simulink model "ASV1_P_RobotMobile1D"  (R2023b)
settings: Solver=VariableStepAuto  StartTime=0.0  StopTime=30  RelTol=1e-3
libraries: simulink x1
settings Model: Creator=LENOVO  LastModifiedBy=LENOVO

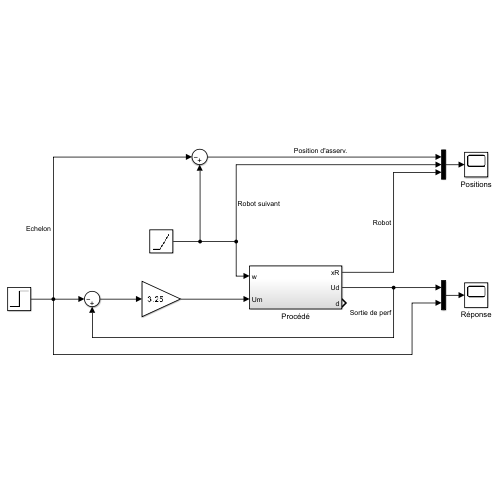
[thumbnail: Simulink's stored preview of the top-level diagram]
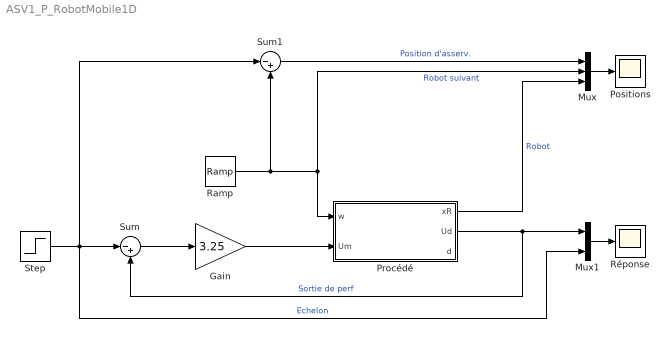
== system ASV1_P_RobotMobile1D ==
  Gain : Gain  Gain=3.25
  Mux : Mux  Inputs=3
  Mux1 : Mux  Inputs=2
  Positions : Scope
  Procédé : Subsystem
  Ramp : simulink/Sources/Ramp  slope=0.5  start=10  InitialOutput=0
  Réponse : Scope
  Step : Step  Time=0  After=0.25  SampleTime=0
  Sum : Sum  Inputs=|-+
  Sum1 : Sum  Inputs=|-+
  wires:
  Step/1 -> Mux1/2, Sum1/1, Sum/1  "Echelon"
  Sum/1 -> Gain/1
  Ramp/1 -> Mux/2, Procédé/1(w), Sum1/2  "Robot suivant"
  Mux/1 -> Positions/1
  Gain/1 -> Procédé/2(Um)
  Sum1/1 -> Mux/1  "Position d'asserv."
  Procédé/1(xR) -> Mux/3  "Robot"
  Procédé/2(Ud) -> Sum/2, Mux1/1  "Sortie de perf"
  Mux1/1 -> Réponse/1

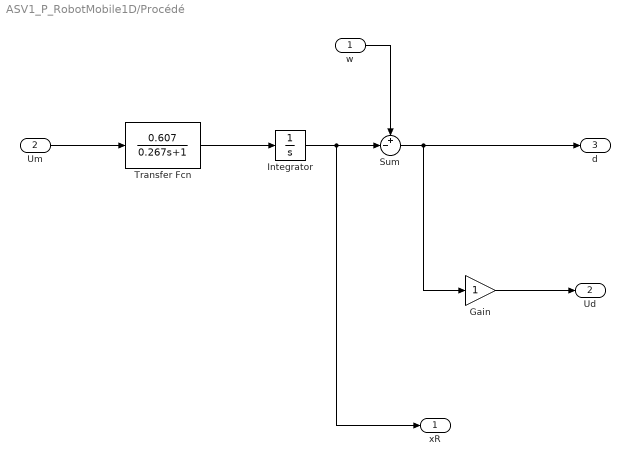
== system ASV1_P_RobotMobile1D/Procédé ==
  w : Inport
  Um : Inport  Port=2
  Gain : Gain
  Integrator : Integrator  InitialCondition=-1
  Sum : Sum  Inputs=+-|
  Transfer Fcn : TransferFcn  Numerator=[0.607]  Denominator=[0.267 1]
  xR : Outport
  Ud : Outport  Port=2
  d : Outport  Port=3
  wires:
  Um/1 -> Transfer Fcn/1
  Integrator/1 -> xR/1, Sum/2
  Sum/1 -> d/1, Gain/1
  Gain/1 -> Ud/1
  Transfer Fcn/1 -> Integrator/1
  w/1 -> Sum/1
